simulink model "FLCU_Gauging"  (R2019b)
settings: Solver=FixedStepAuto  StartTime=0.0  StopTime=10  FixedStep=0.02  RelTol=1e-3
undefined symbols (not defined in the file): alpha, Ca_default_value, Ca_max, Ca_min, Clausius_A, Clausius_B, Density_default_value, Density_max, Density_min, Mass_max, Mass_min, P_default_value, P_max, P_min, T_default_value, T_max, T_min, teta_Ak, teta_Bk, Vp_max, Vp_min
libraries: simulink x2
settings Model: DataDictionary=FLCU_Gauging.sldd  OrderedModelArguments=off  Creator=khato  LastModifiedBy=aymanouchker
settings DataIOCC: ExternalInput=input_data  SignalLoggingName=BusData
settings OptimizationCC: DefaultParameterBehavior=Inlined  UseDivisionForNetSlopeComputation=on  GainParamInheritBuiltInType=on  UseFloatMulNetSlope=on  DefaultUnderspecifiedDataType=single  UseSpecifiedMinMax=on  InlineInvariantSignals=on  EnhancedBackFolding=on  CachingGlobalReferences=on  PassReuseOutputArgsAs=Individual arguments  StateBitsets=on  DataBitsets=on  ZeroExternalMemoryAtStartup=off  ZeroInternalMemoryAtStartup=off  NoFixptDivByZeroProtection=on  EfficientFloat2IntCast=on  LifeSpan=inf  OptimizeBlockOrder=speed  DifferentSizesBufferReuse=on  EfficientTunableParamExpr=on
settings DebuggingCC: SignalInfNanChecking=warning  IntegerOverflowMsg=error  ParameterTunabilityLossMsg=error  UniqueDataStoreMsg=error  AssertControl=DisableAll  StrictBusMsg=ErrorOnBusTreatedAsVector  SFUndirectedBroadcastEventsDiag=error
settings HardwareCC: ProdBitPerLong=64  ProdHWDeviceType=Intel->x86-64 (Mac OS X)
settings SFSimCC: CompileTimeRecursionLimit=0  EnableRuntimeRecursion=off  MATLABDynamicMemAlloc=off
settings RTWCC: SystemTargetFile=ert.tlc  TemplateMakefile=ert_default_tmf  GenerateReport=on  BuildConfiguration=Faster Runs  IncludeHyperlinkInReport=on  LaunchReport=on  GenerateTraceInfo=on  GenerateTraceReport=on  GenerateTraceReportSl=on  GenerateTraceReportSf=on  GenerateTraceReportEml=on
settings CodeAppCC: ForceParamTrailComments=on  IgnoreCustomStorageClasses=off  IgnoreTestpoints=on  OperatorAnnotations=on  SimulinkDataObjDesc=on  SFDataObjDesc=on  MATLABFcnDesc=on  InsertBlockDesc=on  StateflowObjectComments=on  MATLABSourceComments=on  EnableCustomComments=on  ReqsInCode=on
settings ERTTargetCC: TargetLangStandard=C99 (ISO)  UtilityFuncGeneration=Shared location  GenerateSampleERTMain=on  CombineSignalStateStructs=on  SuppressErrorStatus=on  SupportAbsoluteTime=off  MultiInstanceERTCode=on  CodeInterfacePackaging=Reusable function  SupportNonFinite=off  ParenthesesLevel=Maximum  CastingMode=Standards  GenerateSharedConstants=off  InlinedParameterPlacement=NonHierarchical  ERTCustomFileTemplate=example_file_process.tlc  PreserveExpressionOrder=on  PreserveIfCondition=on  EnableSignedLeftShifts=off  EnableSignedRightShifts=off

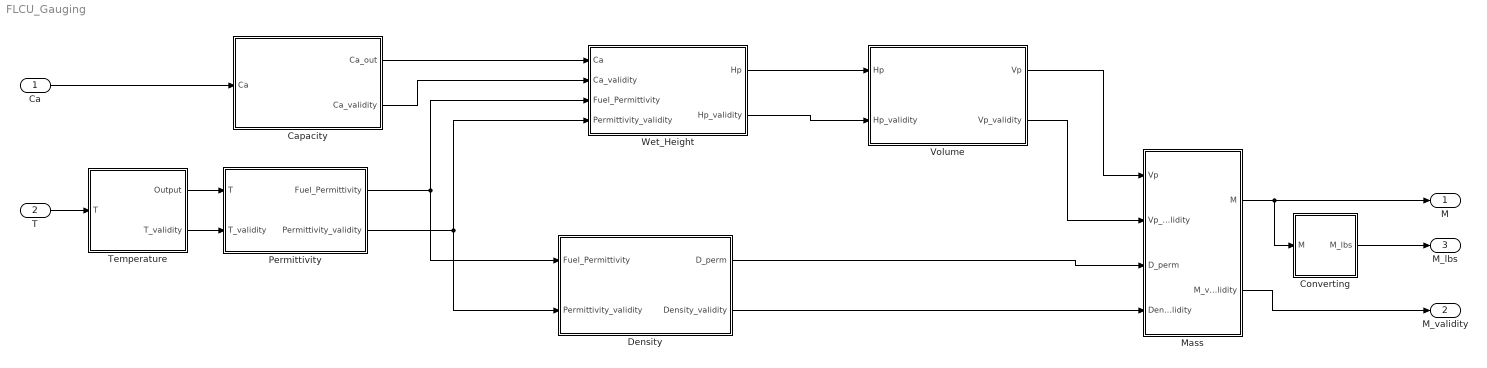
== system FLCU_Gauging ==
  Ca : Inport  OutMin=-10  OutMax=1000  OutDataTypeStr=double  Unit=pF
  T : Inport  Port=2  OutMin=-100  OutMax=150  OutDataTypeStr=double  Unit=°C
  Capacity : Subsystem  TreatAsAtomicUnit=on
      settings: RTWFcnNameOpts=Use subsystem name  RTWFileNameOpts=Use subsystem name
  Converting : Subsystem  TreatAsAtomicUnit=on
      settings: RTWFcnNameOpts=Use subsystem name  RTWFileNameOpts=Use subsystem name
  Density : Subsystem  TreatAsAtomicUnit=on
      settings: RTWFcnNameOpts=Use subsystem name  RTWFileNameOpts=Use subsystem name
  Mass : Subsystem  TreatAsAtomicUnit=on
      settings: RTWFcnNameOpts=Use subsystem name  RTWFileNameOpts=Use subsystem name
  Permittivity : Subsystem  TreatAsAtomicUnit=on
      settings: RTWFcnNameOpts=Use subsystem name  RTWFileNameOpts=Use subsystem name
  Temperature : Subsystem  TreatAsAtomicUnit=on
      settings: RTWFcnNameOpts=Use subsystem name
  Volume : Subsystem  TreatAsAtomicUnit=on
      settings: RTWFcnNameOpts=Use subsystem name  RTWFileNameOpts=Use subsystem name
  Wet_Height : Subsystem  TreatAsAtomicUnit=on
      settings: RTWFcnNameOpts=Use subsystem name  RTWFileNameOpts=Use subsystem name
  M : Outport  OutDataTypeStr=double  Unit=kg
  M_validity : Outport  Port=2  OutDataTypeStr=boolean
  M_lbs : Outport  Port=3  OutDataTypeStr=double  Unit=lb
  wires:
  Temperature/1(Output) -> Permittivity/1(T)
  Capacity/1(Ca_out) -> Wet_Height/1(Ca)
  Permittivity/1(Fuel_Permittivity) -> Density/1(Fuel_Permittivity), Wet_Height/3(Fuel_Permittivity)
  Permittivity/2(Permittivity_validity) -> Wet_Height/4(Permittivity_validity), Density/2(Permittivity_validity)
  Capacity/2(Ca_validity) -> Wet_Height/2(Ca_validity)
  Wet_Height/1(Hp) -> Volume/1(Hp)
  Wet_Height/2(Hp_validity) -> Volume/2(Hp_validity)
  Volume/1(Vp) -> Mass/1(Vp)
  Volume/2(Vp_validity) -> Mass/2(Vp_validity)
  Density/1(D_perm) -> Mass/3(D_perm)
  Density/2(Density_validity) -> Mass/4(Density_validity)
  Mass/1(M) -> Converting/1(M), M/1
  Mass/2(M_validity) -> M_validity/1
  Converting/1(M_lbs) -> M_lbs/1
  Temperature/2(T_validity) -> Permittivity/2(T_validity)
  Ca/1 -> Capacity/1(Ca)
  T/1 -> Temperature/1(T)

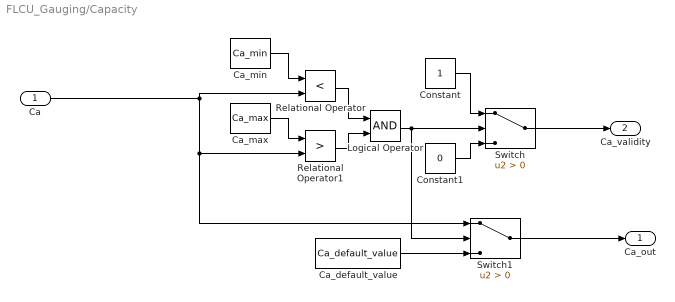
== system FLCU_Gauging/Capacity ==
  Ca : Inport
  Ca_default_value : Constant  Value=Ca_default_value  OutDataTypeStr=double
  Ca_max : Constant  Value=Ca_max  OutDataTypeStr=double
  Ca_min : Constant  Value=Ca_min  OutDataTypeStr=double
  Constant : Constant  OutDataTypeStr=boolean
  Constant1 : Constant  Value=0  OutDataTypeStr=boolean
  Logical Operator : Logic  AllPortsSameDT=off  OutDataTypeStr=boolean
  Relational Operator : RelationalOperator  Operator=<  OutDataTypeStr=boolean  RndMeth=Simplest
  Relational Operator1 : RelationalOperator  Operator=>  OutDataTypeStr=boolean  RndMeth=Simplest
  Switch : Switch  Criteria=u2 > Threshold  OutDataTypeStr=boolean
  Switch1 : Switch  Criteria=u2 > Threshold
  Ca_out : Outport
  Ca_validity : Outport  Port=2
  wires:
  Constant1/1 -> Switch/3
  Logical Operator/1 -> Switch1/2, Switch/2
  Ca/1 -> Relational Operator/2, Relational Operator1/2, Switch1/1
  Constant/1 -> Switch/1
  Relational Operator1/1 -> Logical Operator/2
  Ca_min/1 -> Relational Operator/1
  Switch1/1 -> Ca_out/1
  Ca_default_value/1 -> Switch1/3
  Relational Operator/1 -> Logical Operator/1
  Ca_max/1 -> Relational Operator1/1
  Switch/1 -> Ca_validity/1

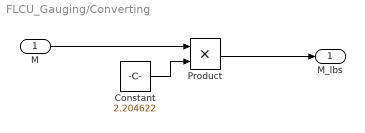
== system FLCU_Gauging/Converting ==
  M : Inport  OutDataTypeStr=double  Unit=kg
  Constant : Constant  Value=2.204622  OutDataTypeStr=double
  Product : Product
  M_lbs : Outport  OutDataTypeStr=double  Unit=lb
  wires:
  Constant/1 -> Product/2
  Product/1 -> M_lbs/1
  M/1 -> Product/1

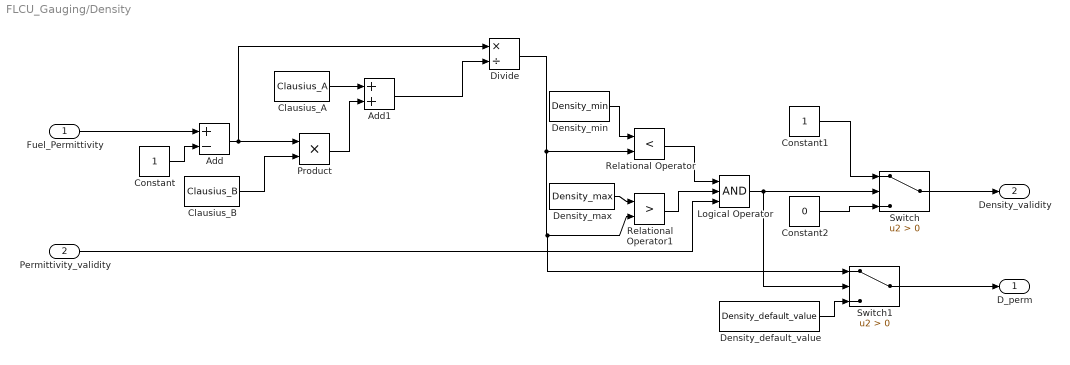
== system FLCU_Gauging/Density ==
  Fuel_Permittivity : Inport  OutDataTypeStr=double
  Permittivity_validity : Inport  Port=2  OutDataTypeStr=boolean
  Add : Sum  Inputs=+-
  Add1 : Sum
  Clausius_A : Constant  Value=Clausius_A  OutMin=0.75  OutMax=1.25  OutDataTypeStr=double
  Clausius_B : Constant  Value=Clausius_B  OutMin=0.25  OutMax=0.5  OutDataTypeStr=double
  Constant : Constant
  Constant1 : Constant  OutDataTypeStr=boolean
  Constant2 : Constant  Value=0  OutDataTypeStr=boolean
  Density_default_value : Constant  Value=Density_default_value  OutMin=0.5  OutMax=1.0  OutDataTypeStr=double
  Density_max : Constant  Value=Density_max  OutDataTypeStr=double
  Density_min : Constant  Value=Density_min  OutDataTypeStr=double
  Divide : Product  Inputs=*/
  Logical Operator : Logic  Inputs=3  AllPortsSameDT=off  OutDataTypeStr=boolean
  Product : Product  OutDataTypeStr=double
  Relational Operator : RelationalOperator  Operator=<  OutDataTypeStr=boolean  RndMeth=Simplest
  Relational Operator1 : RelationalOperator  Operator=>  OutDataTypeStr=boolean  RndMeth=Simplest
  Switch : Switch  Criteria=u2 > Threshold  OutDataTypeStr=boolean
  Switch1 : Switch  Criteria=u2 > Threshold
  D_perm : Outport  OutDataTypeStr=double  Unit=kg/L
  Density_validity : Outport  Port=2  OutDataTypeStr=boolean
  wires:
  Add/1 -> Product/1, Divide/1
  Product/1 -> Add1/2
  Add1/1 -> Divide/2
  Clausius_B/1 -> Product/2
  Clausius_A/1 -> Add1/1
  Constant/1 -> Add/2
  Fuel_Permittivity/1 -> Add/1
  Constant1/1 -> Switch/1
  Logical Operator/1 -> Switch1/2, Switch/2
  Relational Operator/1 -> Logical Operator/1
  Permittivity_validity/1 -> Logical Operator/3
  Relational Operator1/1 -> Logical Operator/2
  Density_default_value/1 -> Switch1/3
  Switch1/1 -> D_perm/1
  Divide/1 -> Switch1/1, Relational Operator1/2, Relational Operator/2
  Constant2/1 -> Switch/3
  Density_min/1 -> Relational Operator/1
  Density_max/1 -> Relational Operator1/1
  Switch/1 -> Density_validity/1

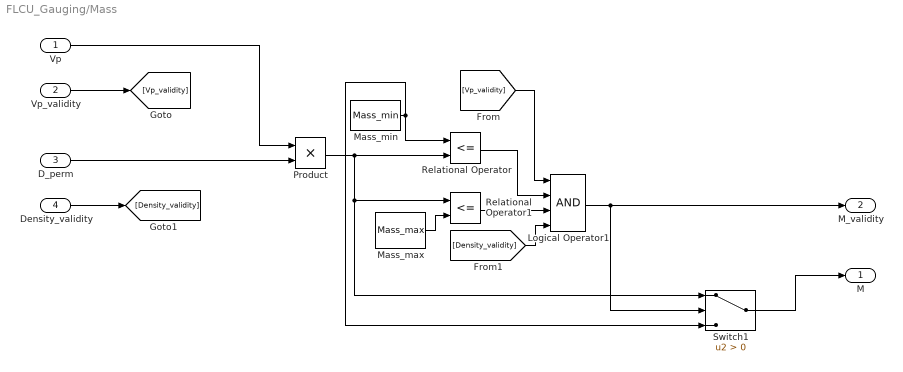
== system FLCU_Gauging/Mass ==
  Vp : Inport  OutDataTypeStr=double  Unit=L
  Vp_validity : Inport  Port=2  OutDataTypeStr=boolean
  D_perm : Inport  Port=3  OutDataTypeStr=double  Unit=kg/L
  Density_validity : Inport  Port=4  OutDataTypeStr=boolean
  Logical Operator1 : Logic  Inputs=4  AllPortsSameDT=off  OutDataTypeStr=boolean
  Mass_max : Constant  Value=Mass_max  OutDataTypeStr=double
  Mass_min : Constant  Value=Mass_min  OutDataTypeStr=double
  Product : Product
  Relational Operator : RelationalOperator  Operator=<=  OutDataTypeStr=boolean  RndMeth=Simplest
  Relational Operator1 : RelationalOperator  Operator=<=  OutDataTypeStr=boolean  RndMeth=Simplest
  Switch1 : Switch  Criteria=u2 > Threshold
  M : Outport  OutDataTypeStr=double  Unit=kg
  M_validity : Outport  Port=2  OutDataTypeStr=boolean
  wires:
  Product/1 -> Relational Operator1/1, Switch1/1, Relational Operator/2
  [Vp_validity] -> Logical Operator1/1
  Mass_max/1 -> Relational Operator1/2
  [Density_validity] -> Logical Operator1/4
  Switch1/1 -> M/1
  Logical Operator1/1 -> M_validity/1, Switch1/2
  Relational Operator/1 -> Logical Operator1/2
  Mass_min/1 -> Switch1/3, Relational Operator/1
  Relational Operator1/1 -> Logical Operator1/3
  Density_validity/1 -> [Density_validity]
  Vp_validity/1 -> [Vp_validity]
  D_perm/1 -> Product/2
  Vp/1 -> Product/1

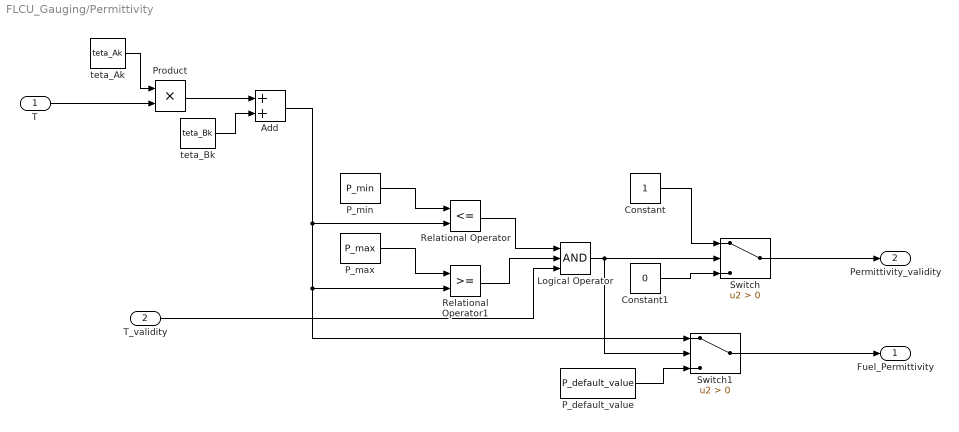
== system FLCU_Gauging/Permittivity ==
  T : Inport  OutDataTypeStr=double  Unit=°C
  T_validity : Inport  Port=2  OutMin=0  OutMax=1  OutDataTypeStr=boolean
  Add : Sum  AccumDataTypeStr=double  OutDataTypeStr=double
  Constant : Constant  OutDataTypeStr=boolean
  Constant1 : Constant  Value=0  OutDataTypeStr=boolean
  Logical Operator : Logic  Inputs=3  AllPortsSameDT=off  OutDataTypeStr=boolean
  P_default_value : Constant  Value=P_default_value  OutDataTypeStr=double
  P_max : Constant  Value=P_max  OutDataTypeStr=double
  P_min : Constant  Value=P_min  OutDataTypeStr=double
  Product : Product  OutDataTypeStr=double
  Relational Operator : RelationalOperator  Operator=<=  OutDataTypeStr=boolean  RndMeth=Simplest
  Relational Operator1 : RelationalOperator  OutDataTypeStr=boolean  RndMeth=Simplest
  Switch : Switch  Criteria=u2 > Threshold  OutDataTypeStr=boolean
  Switch1 : Switch  Criteria=u2 > Threshold
  teta_Ak : Constant  Value=teta_Ak  OutMin=1.8  OutMax=2.5  OutDataTypeStr=double
  teta_Bk : Constant  Value=teta_Bk  OutMin=-0.1  OutMax=0  OutDataTypeStr=double
  Fuel_Permittivity : Outport  OutDataTypeStr=double
  Permittivity_validity : Outport  Port=2  OutDataTypeStr=boolean
  wires:
  Product/1 -> Add/1
  teta_Bk/1 -> Add/2
  T/1 -> Product/2
  teta_Ak/1 -> Product/1
  P_min/1 -> Relational Operator/1
  P_max/1 -> Relational Operator1/1
  Relational Operator/1 -> Logical Operator/1
  Relational Operator1/1 -> Logical Operator/2
  T_validity/1 -> Logical Operator/3
  Logical Operator/1 -> Switch1/2, Switch/2
  Switch/1 -> Permittivity_validity/1
  Switch1/1 -> Fuel_Permittivity/1
  Constant/1 -> Switch/1
  Constant1/1 -> Switch/3
  P_default_value/1 -> Switch1/3
  Add/1 -> Switch1/1, Relational Operator1/2, Relational Operator/2

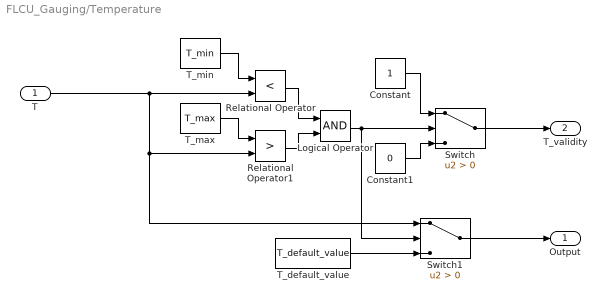
== system FLCU_Gauging/Temperature ==
  T : Inport  OutDataTypeStr=double  Unit=°C
  Constant : Constant  OutDataTypeStr=boolean
  Constant1 : Constant  Value=0  OutDataTypeStr=boolean
  Logical Operator : Logic  AllPortsSameDT=off  OutDataTypeStr=boolean
  Relational Operator : RelationalOperator  Operator=<  OutDataTypeStr=boolean  RndMeth=Simplest
  Relational Operator1 : RelationalOperator  Operator=>  OutDataTypeStr=boolean  RndMeth=Simplest
  Switch : Switch  Criteria=u2 > Threshold  OutDataTypeStr=boolean
  Switch1 : Switch  Criteria=u2 > Threshold
  T_default_value : Constant  Value=T_default_value  OutDataTypeStr=double
  T_max : Constant  Value=T_max  OutDataTypeStr=double
  T_min : Constant  Value=T_min  OutDataTypeStr=double
  Output : Outport  OutDataTypeStr=double  Unit=°C
  T_validity : Outport  Port=2  OutMin=0  OutMax=1  OutDataTypeStr=boolean
  wires:
  T_default_value/1 -> Switch1/3
  Constant1/1 -> Switch/3
  Relational Operator1/1 -> Logical Operator/2
  T_min/1 -> Relational Operator/1
  Constant/1 -> Switch/1
  T/1 -> Relational Operator1/2, Switch1/1, Relational Operator/2
  Switch1/1 -> Output/1
  Relational Operator/1 -> Logical Operator/1
  Logical Operator/1 -> Switch1/2, Switch/2
  Switch/1 -> T_validity/1
  T_max/1 -> Relational Operator1/1

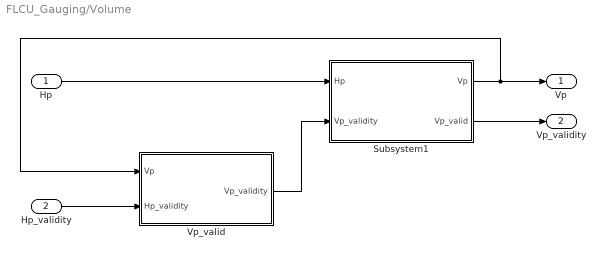
== system FLCU_Gauging/Volume ==
  Hp : Inport  OutDataTypeStr=double
  Hp_validity : Inport  Port=2  OutDataTypeStr=boolean
  Subsystem1 : Subsystem
  Vp_valid : Subsystem
  Vp : Outport  OutDataTypeStr=double  Unit=l
  Vp_validity : Outport  Port=2  OutDataTypeStr=boolean
  wires:
  Hp_validity/1 -> Vp_valid/2(Hp_validity)
  Hp/1 -> Subsystem1/1(Hp)
  Subsystem1/1(Vp) -> Vp_valid/1(Vp), Vp/1
  Vp_valid/1(Vp_validity) -> Subsystem1/2(Vp_validity)
  Subsystem1/2(Vp_valid) -> Vp_validity/1

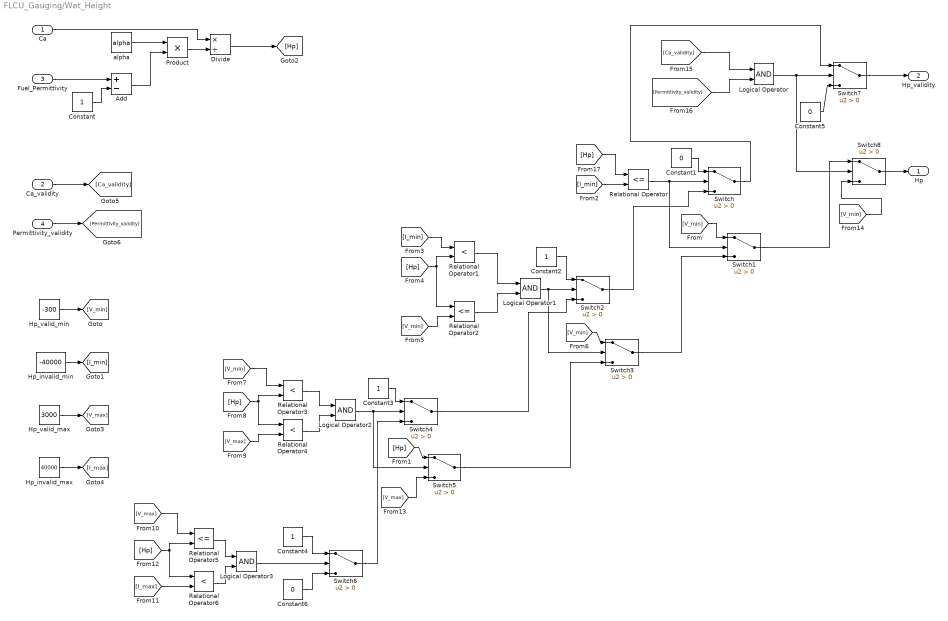
== system FLCU_Gauging/Wet_Height ==
  Ca : Inport  OutDataTypeStr=double  Unit=pF
  Ca_validity : Inport  Port=2  OutDataTypeStr=boolean
  Fuel_Permittivity : Inport  Port=3  OutDataTypeStr=double
  Permittivity_validity : Inport  Port=4  OutDataTypeStr=boolean
  Add : Sum  Inputs=+-
  Constant : Constant
  Constant1 : Constant  Value=0  OutDataTypeStr=boolean
  Constant2 : Constant  OutDataTypeStr=boolean
  Constant3 : Constant  OutDataTypeStr=boolean
  Constant4 : Constant  OutDataTypeStr=boolean
  Constant5 : Constant  Value=0  OutDataTypeStr=boolean
  Constant6 : Constant  Value=0  OutDataTypeStr=boolean
  Divide : Product  Inputs=*/
  Hp_invalid_max : Constant  Value=40000  OutDataTypeStr=double
  Hp_invalid_min : Constant  Value=-40000  OutDataTypeStr=double
  Hp_valid_max : Constant  Value=3000  OutDataTypeStr=double
  Hp_valid_min : Constant  Value=-300  OutDataTypeStr=double
  Logical Operator{,1..3} (4 alike) : Logic  AllPortsSameDT=off  OutDataTypeStr=boolean
  Product : Product  OutDataTypeStr=double
  Relational Operator : RelationalOperator  Operator=<=  OutDataTypeStr=boolean  RndMeth=Simplest
  Relational Operator{1,3..4,6} (4 alike) : RelationalOperator  Operator=<  OutDataTypeStr=boolean  RndMeth=Simplest
  Relational Operator2 : RelationalOperator  Operator=<=  OutDataTypeStr=boolean  RndMeth=Simplest
  Relational Operator5 : RelationalOperator  Operator=<=  OutDataTypeStr=boolean  RndMeth=Simplest
  Switch{,2,4,6..7} (5 alike) : Switch  Criteria=u2 > Threshold  OutDataTypeStr=boolean
  Switch{1,3,5,8} (4 alike) : Switch  Criteria=u2 > Threshold
  alpha : Constant  Value=alpha  OutMin=0.01  OutMax=0.3  OutDataTypeStr=double
  Hp : Outport  OutDataTypeStr=double  Unit=mm
  Hp_validity : Outport  Port=2  OutDataTypeStr=boolean
  wires:
  Logical Operator3/1 -> Switch6/2
  Permittivity_validity/1 -> [Permittivity_validity]
  Ca/1 -> Divide/1
  [V_min] -> Switch8/3
  Constant5/1 -> Switch7/3
  Divide/1 -> [Hp]
  alpha/1 -> Product/1
  Add/1 -> Product/2
  Product/1 -> Divide/2
  Constant/1 -> Add/2
  Fuel_Permittivity/1 -> Add/1
  [Ca_validity] -> Logical Operator/1
  [Permittivity_validity] -> Logical Operator/2
  Relational Operator/1 -> Switch1/2, Switch/2
  Constant1/1 -> Switch/1
  Hp_valid_min/1 -> [V_min]
  [V_min] -> Switch1/1
  Hp_invalid_min/1 -> [I_min]
  [I_min] -> Relational Operator/2
  [I_min] -> Relational Operator1/1
  [Hp] -> Relational Operator2/1, Relational Operator1/2
  [V_min] -> Relational Operator2/2
  Relational Operator1/1 -> Logical Operator1/1
  Relational Operator2/1 -> Logical Operator1/2
  Logical Operator1/1 -> Switch3/2, Switch2/2
  Constant2/1 -> Switch2/1
  Switch2/1 -> Switch/3
  [V_min] -> Switch3/1
  Switch3/1 -> Switch1/3
  Hp_valid_max/1 -> [V_max]
  Hp_invalid_max/1 -> [I_max]
  [V_min] -> Relational Operator3/1
  [Hp] -> Relational Operator4/1, Relational Operator3/2
  [V_max] -> Relational Operator4/2
  Relational Operator3/1 -> Logical Operator2/1
  Relational Operator4/1 -> Logical Operator2/2
  Logical Operator2/1 -> Switch5/2, Switch4/2
  Constant3/1 -> Switch4/1
  [Hp] -> Switch5/1
  Switch4/1 -> Switch2/3
  Switch5/1 -> Switch3/3
  [V_max] -> Relational Operator5/1
  [Hp] -> Relational Operator5/2, Relational Operator6/1
  [I_max] -> Relational Operator6/2
  Constant4/1 -> Switch6/1
  Relational Operator5/1 -> Logical Operator3/1
  Relational Operator6/1 -> Logical Operator3/2
  Switch6/1 -> Switch4/3
  Constant6/1 -> Switch6/3
  [V_max] -> Switch5/3
  Logical Operator/1 -> Switch8/2, Switch7/2
  Switch/1 -> Switch7/1
  Switch7/1 -> Hp_validity/1
  Switch8/1 -> Hp/1
  Switch1/1 -> Switch8/1
  Ca_validity/1 -> [Ca_validity]
  [Hp] -> Relational Operator/1

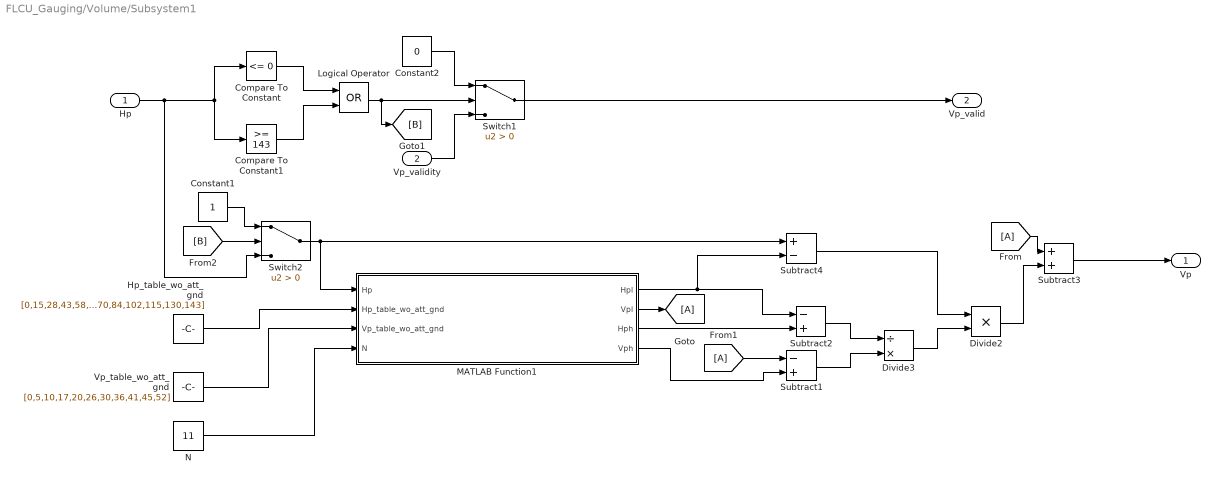
== system FLCU_Gauging/Volume/Subsystem1 ==
  Hp : Inport  OutDataTypeStr=double
  Vp_validity : Inport  Port=2  OutDataTypeStr=boolean
  Compare To Constant : simulink/Logic and Bit Operations/Compare To Constant  relop=<=  const=0  OutDataTypeStr=boolean
  Compare To Constant1 : simulink/Logic and Bit Operations/Compare To Constant  relop=>=  const=143  OutDataTypeStr=boolean
  Constant1 : Constant
  Constant2 : Constant  Value=0  OutDataTypeStr=boolean
  Divide2 : Product  Inputs=**
  Divide3 : Product  Inputs=/*
  Hp_table_wo_att_gnd : Constant  Value=[0,15,28,43,58,70,84,102,115,130,143]  OutDataTypeStr=double
  Logical Operator : Logic  Operator=OR  AllPortsSameDT=off  OutDataTypeStr=boolean
  MATLAB Function1 : MATLAB Function  TreatAsAtomicUnit=on
  N : Constant  Value=11
  Subtract1 : Sum  Inputs=-+
  Subtract2 : Sum  Inputs=-+
  Subtract3 : Sum
  Subtract4 : Sum  Inputs=+-
  Switch1 : Switch  Criteria=u2 > Threshold
  Switch2 : Switch  Criteria=u2 > Threshold
  Vp_table_wo_att_gnd : Constant  Value=[0,5,10,17,20,26,30,36,41,45,52]  OutDataTypeStr=double
  Vp : Outport  OutDataTypeStr=double  Unit=l
  Vp_valid : Outport  Port=2  OutDataTypeStr=boolean
  wires:
  [A] -> Subtract1/1
  Subtract3/1 -> Vp/1
  MATLAB Function1/1(Hpl) -> Subtract4/2, Subtract2/1
  MATLAB Function1/4(Vph) -> Subtract1/2
  Subtract2/1 -> Divide3/1
  MATLAB Function1/2(Vpl) -> [A]
  N/1 -> MATLAB Function1/4(N)
  Subtract4/1 -> Divide2/1
  Divide3/1 -> Divide2/2
  Subtract1/1 -> Divide3/2
  [A] -> Subtract3/1
  MATLAB Function1/3(Hph) -> Subtract2/2
  Divide2/1 -> Subtract3/2
  Hp_table_wo_att_gnd/1 -> MATLAB Function1/2(Hp_table_wo_att_gnd)
  Vp_table_wo_att_gnd/1 -> MATLAB Function1/3(Vp_table_wo_att_gnd)
  Hp/1 -> Switch2/3, Compare To Constant1/1, Compare To Constant/1
  Compare To Constant/1 -> Logical Operator/1
  Compare To Constant1/1 -> Logical Operator/2
  Logical Operator/1 -> [B], Switch1/2
  Constant2/1 -> Switch1/1
  Switch1/1 -> Vp_valid/1
  Vp_validity/1 -> Switch1/3
  Constant1/1 -> Switch2/1
  [B] -> Switch2/2
  Switch2/1 -> MATLAB Function1/1(Hp), Subtract4/1

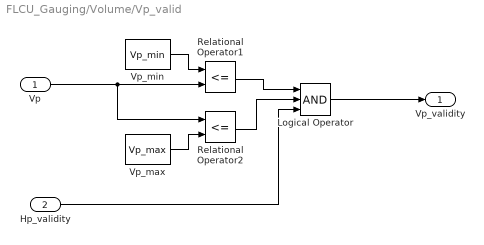
== system FLCU_Gauging/Volume/Vp_valid ==
  Vp : Inport
  Hp_validity : Inport  Port=2
  Logical Operator : Logic  Inputs=3  AllPortsSameDT=off  OutDataTypeStr=boolean
  Relational Operator1 : RelationalOperator  Operator=<=  OutDataTypeStr=boolean  RndMeth=Simplest
  Relational Operator2 : RelationalOperator  Operator=<=  OutDataTypeStr=boolean  RndMeth=Simplest
  Vp_max : Constant  Value=Vp_max
  Vp_min : Constant  Value=Vp_min  OutDataTypeStr=double
  Vp_validity : Outport
  wires:
  Relational Operator2/1 -> Logical Operator/2
  Vp_max/1 -> Relational Operator2/2
  Logical Operator/1 -> Vp_validity/1
  Vp/1 -> Relational Operator1/2, Relational Operator2/1
  Vp_min/1 -> Relational Operator1/1
  Hp_validity/1 -> Logical Operator/3
  Relational Operator1/1 -> Logical Operator/1

== matlab function FLCU_Gauging/Volume/Subsystem1/MATLAB Function1 ==
  data: Hp input; Hp_table_wo_att_gnd input; Vp_table_wo_att_gnd input; Hpl output; N input; Vpl output; Hph output; Vph output
function [Hpl, Vpl, Hph, Vph] = findClosestSuppInf(Hp,Hp_table_wo_att_gnd,Vp_table_wo_att_gnd,N)
%%Corner cases
i=2;
        while(i<=N && Hp_table_wo_att_gnd(i)< Hp)
            i=i+1;
        end
        if(Hp_table_wo_att_gnd(i) == Hp)
            Hpl=Hp_table_wo_att_gnd(i);
            Hph=Hp_table_wo_att_gnd(i);
            Vpl=Vp_table_wo_att_gnd(i);
            Vph=Vp_table_wo_att_gnd(i);
        else
            Hpl=Hp_table_wo_att_gnd(i-1);
            Hph=Hp_table_wo_att_gnd(i);
            Vpl=Vp_table_wo_att_gnd(i-1);
            Vph=Vp_table_wo_att_gnd(i);
        end
 end
